simulink model "zn"  (R2022b)
settings: Solver=VariableStepAuto  StartTime=0.0  StopTime=10.0  RelTol=1e-3
settings Model: Creator=IdeaPad 700  LastModifiedBy=IdeaPad 700

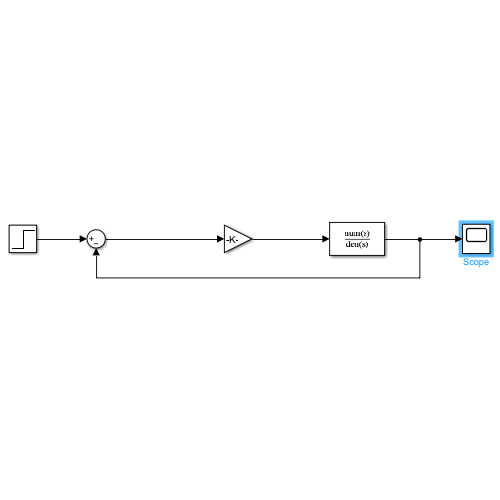
[thumbnail: Simulink's stored preview of the top-level diagram]
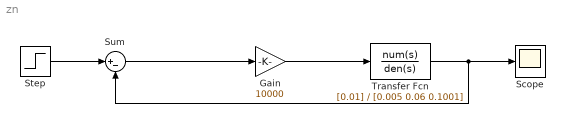
== system zn ==
  Gain : Gain  Gain=10000
  Scope : Scope
  Step : Step  SampleTime=0
  Sum : Sum  Inputs=|+-
  Transfer Fcn : TransferFcn  Numerator=[0.01]  Denominator=[0.005 0.06 0.1001]
  wires:
  Step/1 -> Sum/1
  Sum/1 -> Gain/1
  Gain/1 -> Transfer Fcn/1
  Transfer Fcn/1 -> Sum/2, Scope/1
